simulink model "DelayStateMachine"  (R2022b)
settings: Solver=VariableStepAuto  StartTime=0.0  StopTime=10.0  RelTol=1e-3
settings Model: Creator=salman  LastModifiedBy=salman

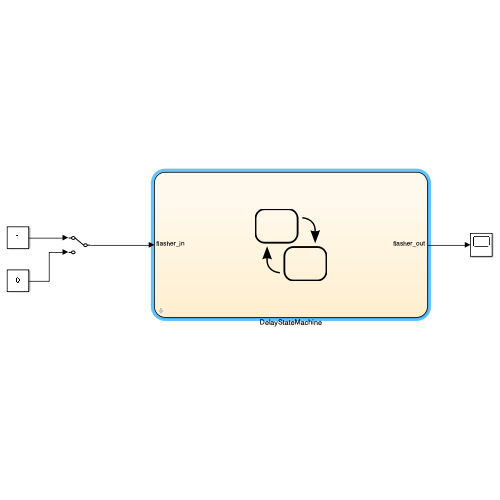
[thumbnail: Simulink's stored preview of the top-level diagram]
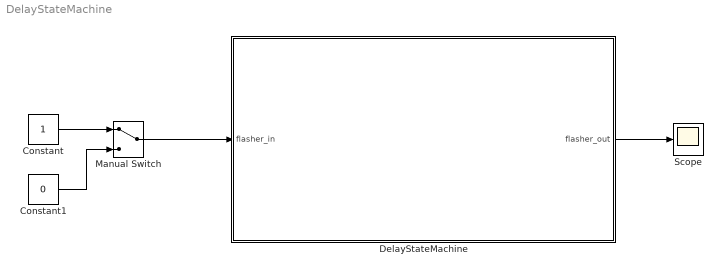
== system DelayStateMachine ==
  Constant : Constant
  Constant1 : Constant  Value=0
  DelayStateMachine : Stateflow chart  TreatAsAtomicUnit=on  mask{delay=10}
      mask prompts: delay "Enter Delay Time"
  Manual Switch : ManualSwitch
  Scope : Scope
  wires:
  Manual Switch/1 -> DelayStateMachine/1(flasher_in)
  Constant/1 -> Manual Switch/1
  Constant1/1 -> Manual Switch/2
  DelayStateMachine/1(flasher_out) -> Scope/1

== stateflow chart DelayStateMachine/DelayStateMachine ==
  state Idle
    entry:
    flasher_out = 0;
  state OFF
    entry:
    flasher_out=0;
  state ON
    entry:
    flasher_out = 1;
  (default) -> Idle
  Idle -> ON : [flasher_in==1]
  OFF -> Idle [order 2] : [flasher_in == 0]
  ON -> OFF : [after(delay,sec) || flasher_in == 0]
  OFF -> ON [order 1] : [after(delay,sec) && flasher_in ==1]
  data: flasher_in input; flasher_out output; delay parameter
